simulink model "simulation_vex"  (R2024a)
settings: Solver=FixedStepAuto  StartTime=0.0  StopTime=100.0  RelTol=1e-3  EnableMultiTasking=on
libraries: vexarmcortexlib x33
settings Model: ExtModeTrigDuration=25  Creator=Mattie  LastModifiedBy=Monarch Robotics
settings SolverCC: AutoInsertRateTranBlk=on
settings OptimizationCC: EnhancedBackFolding=on  PassReuseOutputArgsAs=Individual arguments  ZeroExternalMemoryAtStartup=off  ZeroInternalMemoryAtStartup=off  MaxStackSize=64  OptimizeBlockOrder=speed  DifferentSizesBufferReuse=on  OptimizationCustomize=off  EfficientTunableParamExpr=on
settings DebuggingCC: ParameterTunabilityLossMsg=error
settings HardwareCC: ProdBitPerPointer=32  ProdBitPerSizeT=32  ProdBitPerPtrDiffT=32  ProdLargestAtomicInteger=Long  ProdLargestAtomicFloat=Double  ProdWordSize=32  ProdHWDeviceType=ARM Compatible->ARM Cortex
settings SFSimCC: MATLABDynamicMemAlloc=off
settings RTWCC: Description=Embedded Coder  SystemTargetFile=ert.tlc  HardwareBoard=ARM Cortex-based VEX Microcontroller  TLCOptions="-aInlineSetEventsForThisBaseRateFcn=TLC_FALSE -aSuppressMultiTaskScheduler=TLC_FALSE  -aRateBasedStepFcn=0"  TemplateMakefile=ert_default_tmf  Toolchain=GNU Tools for VEX ARM Cortex
settings CodeAppCC: ForceParamTrailComments=on  IgnoreCustomStorageClasses=off  OperatorAnnotations=on  SimulinkDataObjDesc=on  SFDataObjDesc=on  InsertBlockDesc=on
settings ERTTargetCC: ExtModeTransport=1  ExtModeMexFile=ext_serial_win32_comm

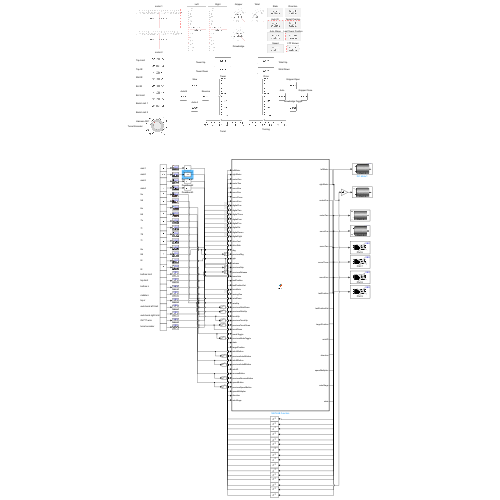
[thumbnail: Simulink's stored preview of the top-level diagram]
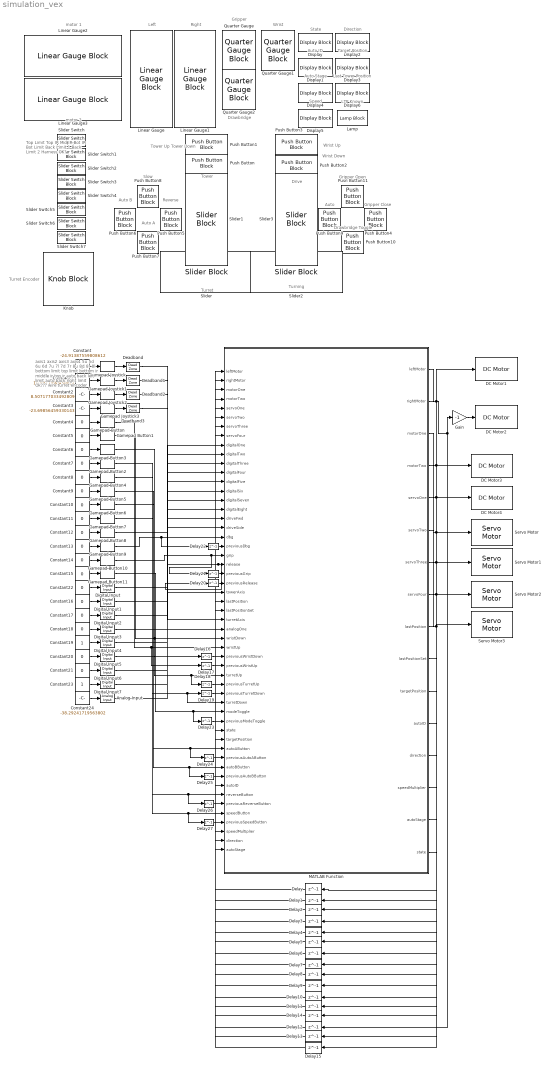
== system simulation_vex ==
  note: State
  note: Drawbridge
  note: Wrist
  note: Gripper
  note: Right
  note: Left
  note: motor 2
  note: motor 1
  note: Turret Encoder
  note: Top Limit
      |
      |
      | Top IR
      |
      |
      | Mid IR
      |
      |
      | Bot IR
      |
      |
      | Bot Limit
      |
      |
      | Back Limit 1
      |
      |
      | Back Limit 2
      |
      |
      | Harness OK?
  note: Drive
  note: Tower
  note: Turret
  note: Turning
  note: Gripper Close
  note: Gripper Open
  note: Auto
  note: Slow
  note: Reverse
  note: Auto A
  note: Auto B
  note: Wrist Down
  note: Wrist Up
  note: Tower Up
      |
      |
      | Tower Down
  note: axis1
      |
      | axis2
      |
      | axis3
      |
      |
      | axis4
      |
      | 5u
      |
      | 5d
      |
      |
      | 6u
      |
      | 6d
      |
      | 7u
      |
      |
      | 7l
      |
      | 7d
      |
      | 7r
      |
      |
      | 8u
      |
      | 8d
      |
      | 8r
      |
      |
      | 8l
      |
      | bottom limit
      |
      | top limit
      |
      | bottom ir
      |
      |
      | middle ir
      |
      | top ir
      |
      | auto back left limit
      |
      |
      | auto back right limit
      |
      | Ok??? wire
      |
      | turret encoder
  note: LTP Known
  note: Direction
  note: Target Position
  note: Auto ID
  note: Speed
  note: Auto Stage
  note: Last Tower Position
  note: Drawbridge Toggle
  Analog Input : vexarmcortexlib/Sensors/Analog Input  inChan=1  SimulationIn=on  SampleTime=0.2
  Constant : Constant  Value=-24.91387559808612
  Constant1 : Constant  Value=10.9377990430622
  Constant{4..18,20..22} (18 alike) : Constant  Value=0
  Constant19 : Constant
  Constant2 : Constant  Value=8.507177033492809
  Constant23 : Constant
  Constant24 : Constant  Value=-38.29241719563802
  Constant3 : Constant  Value=-23.69856459330143
  DC Motor1 : vexarmcortexlib/Actuators/DC Motor  motor=2  scaleFactor=1/13.5  SimulationOut=off
  DC Motor2 : vexarmcortexlib/Actuators/DC Motor  motor=3  scaleFactor=1/13.5  SimulationOut=off
  DC Motor3 : vexarmcortexlib/Actuators/DC Motor  motor=4  scaleFactor=1/13.5  SimulationOut=off
  DC Motor4 : vexarmcortexlib/Actuators/DC Motor  motor=5  scaleFactor=1/13.5  SimulationOut=off
  Deadband{,1..3} (4 alike) : DeadZone  LowerValue=-5  UpperValue=5
  Delay{,1..27} (28 alike) : Delay  DelayLength=1
  Digital Input : vexarmcortexlib/Sensors/Digital Input  inChan=1  SimulationIn=on  SampleTime=0.2
  Digital Input1 : vexarmcortexlib/Sensors/Digital Input  inChan=2  SimulationIn=on  SampleTime=0.2
  Digital Input2 : vexarmcortexlib/Sensors/Digital Input  inChan=3  SimulationIn=on  SampleTime=0.2
  Digital Input3 : vexarmcortexlib/Sensors/Digital Input  inChan=4  SimulationIn=on  SampleTime=0.2
  Digital Input4 : vexarmcortexlib/Sensors/Digital Input  inChan=5  SimulationIn=on  SampleTime=0.2
  Digital Input5 : vexarmcortexlib/Sensors/Digital Input  inChan=6  SimulationIn=on  SampleTime=0.2
  Digital Input6 : vexarmcortexlib/Sensors/Digital Input  inChan=7  SimulationIn=on  SampleTime=0.2
  Digital Input7 : vexarmcortexlib/Sensors/Digital Input  inChan=8  SimulationIn=on  SampleTime=0.2
  Display{,1..6} (7 alike) : DisplayBlock  LabelPosition=Hide  Transparency=1
  Gain : Gain  Gain=-1
  Gamepad Button : vexarmcortexlib/Gamepad/Gamepad Button  joystick=1  chan=5  button56=Up  button78=Down  SimulationIn=on  SampleTime=0.02
  Gamepad Button1 : vexarmcortexlib/Gamepad/Gamepad Button  joystick=1  chan=5  button56=Down  button78=Down  SimulationIn=on  SampleTime=0.02
  Gamepad Button10 : vexarmcortexlib/Gamepad/Gamepad Button  joystick=1  chan=8  button56=Up  button78=Right  SimulationIn=on  SampleTime=0.02
  Gamepad Button11 : vexarmcortexlib/Gamepad/Gamepad Button  joystick=1  chan=8  button56=Up  button78=Left  SimulationIn=on  SampleTime=0.02
  Gamepad Button2 : vexarmcortexlib/Gamepad/Gamepad Button  joystick=1  chan=6  button56=Down  button78=Down  SimulationIn=on  SampleTime=0.02
  Gamepad Button3 : vexarmcortexlib/Gamepad/Gamepad Button  joystick=1  chan=6  button56=Up  button78=Down  SimulationIn=on  SampleTime=0.02
  Gamepad Button4 : vexarmcortexlib/Gamepad/Gamepad Button  joystick=1  chan=7  button56=Up  button78=Up  SimulationIn=on  SampleTime=0.02
  Gamepad Button5 : vexarmcortexlib/Gamepad/Gamepad Button  joystick=1  chan=7  button56=Up  button78=Left  SimulationIn=on  SampleTime=0.02
  Gamepad Button6 : vexarmcortexlib/Gamepad/Gamepad Button  joystick=1  chan=7  button56=Up  button78=Down  SimulationIn=on  SampleTime=0.02
  Gamepad Button7 : vexarmcortexlib/Gamepad/Gamepad Button  joystick=1  chan=7  button56=Up  button78=Right  SimulationIn=on  SampleTime=0.02
  Gamepad Button8 : vexarmcortexlib/Gamepad/Gamepad Button  joystick=1  chan=8  button56=Up  button78=Up  SimulationIn=on  SampleTime=0.02
  Gamepad Button9 : vexarmcortexlib/Gamepad/Gamepad Button  joystick=1  chan=8  button56=Up  button78=Down  SimulationIn=on  SampleTime=0.02
  Gamepad Joystick : vexarmcortexlib/Gamepad/Gamepad Joystick  joystick=1  chan=1  SimulationIn=on  SampleTime=0.02
  Gamepad Joystick1 : vexarmcortexlib/Gamepad/Gamepad Joystick  joystick=1  chan=2  SimulationIn=on  SampleTime=0.02
  Gamepad Joystick2 : vexarmcortexlib/Gamepad/Gamepad Joystick  joystick=1  chan=3  SimulationIn=on  SampleTime=0.02
  Gamepad Joystick3 : vexarmcortexlib/Gamepad/Gamepad Joystick  joystick=1  chan=4  SimulationIn=on  SampleTime=0.02
  Knob : KnobBlock  LabelPosition=Hide  ScaleMin=-127  ScaleMax=127
  Lamp : LampBlock  LabelPosition=Hide
  Linear Gauge{,1..3} (4 alike) : LinearGaugeBlock  LabelPosition=Hide  ScaleMin=-127  ScaleMax=127
  MATLAB Function : MATLAB Function  TreatAsAtomicUnit=on
  Push Button{,1..11} (12 alike) : PushButtonBlock  OffValue=0.000000
  Quarter Gauge : QuarterGaugeBlock  LabelPosition=Hide  ScaleMin=-127  ScaleMax=127
  Quarter Gauge1 : QuarterGaugeBlock  LabelPosition=Hide  ScaleMin=-127  ScaleMax=127
  Quarter Gauge2 : QuarterGaugeBlock  LabelPosition=Hide  ScaleMin=-127  ScaleMax=127
  Servo Motor : vexarmcortexlib/Actuators/Servo Motor  motor=6  scaleFactor=60/127  SimulationOut=off
  Servo Motor1 : vexarmcortexlib/Actuators/Servo Motor  motor=7  scaleFactor=60/127  SimulationOut=off
  Servo Motor2 : vexarmcortexlib/Actuators/Servo Motor  motor=8  scaleFactor=60/127  SimulationOut=off
  Servo Motor3 : vexarmcortexlib/Actuators/Servo Motor  motor=9  scaleFactor=60/127  SimulationOut=off
  Slider{,1..3} (4 alike) : SliderBlock  LabelPosition=Hide  ScaleMin=-127  ScaleMax=127
  Slider Switch{,1..7} (8 alike) : SliderSwitchBlock  LabelPosition=Hide
      settings: Values={{'Off', 'On'}, [0 1]}
  wires:
  MATLAB Function/15(autoStage) -> Delay/1
  MATLAB Function/14(speedMultiplier) -> Delay1/1
  MATLAB Function/13(direction) -> Delay2/1
  MATLAB Function/12(autoID) -> Delay3/1
  MATLAB Function/11(targetPosition) -> Delay4/1
  MATLAB Function/10(lastPositionSet) -> Delay5/1
  MATLAB Function/9(lastPosition) -> Delay6/1
  MATLAB Function/8(servoFour) -> Servo Motor3/1, Delay7/1
  MATLAB Function/7(servoThree) -> Servo Motor2/1, Delay8/1
  MATLAB Function/6(servoTwo) -> Servo Motor1/1, Delay9/1
  MATLAB Function/5(servoOne) -> Servo Motor/1, Delay10/1
  MATLAB Function/1(leftMotor) -> DC Motor1/1, Delay13/1
  MATLAB Function/3(motorOne) -> DC Motor3/1, Delay14/1
  MATLAB Function/2(rightMotor) -> Gain/1, Delay12/1
  MATLAB Function/4(motorTwo) -> DC Motor4/1, Delay11/1
  Delay/1 -> MATLAB Function/53("autoStage ")
  Delay1/1 -> MATLAB Function/51("speedMultiplier ")
  Delay2/1 -> MATLAB Function/52("direction ")
  Delay3/1 -> MATLAB Function/46("autoID ")
  Delay4/1 -> MATLAB Function/41("targetPosition ")
  Delay5/1 -> MATLAB Function/27("lastPositionSet ")
  Delay13/1 -> MATLAB Function/1("leftMotor ")
  Delay12/1 -> MATLAB Function/2("rightMotor ")
  Delay14/1 -> MATLAB Function/3("motorOne ")
  Delay11/1 -> MATLAB Function/4("motorTwo ")
  Delay10/1 -> MATLAB Function/5("servoOne ")
  Delay9/1 -> MATLAB Function/6("servoTwo ")
  Delay8/1 -> MATLAB Function/7("servoThree ")
  Delay7/1 -> MATLAB Function/8("servoFour ")
  Delay6/1 -> MATLAB Function/26("lastPosition ")
  Gamepad Joystick/1 -> Deadband/1
  Gamepad Joystick1/1 -> Deadband1/1
  Gamepad Joystick2/1 -> Deadband2/1
  Gamepad Joystick3/1 -> Deadband3/1
  Gamepad Button/1 -> MATLAB Function/31(wristUp), Delay17/1
  Gamepad Button1/1 -> MATLAB Function/30(wristDown), Delay16/1
  Gamepad Button2/1 -> MATLAB Function/37(turretDown), Delay19/1
  Gamepad Button3/1 -> Delay18/1, MATLAB Function/34(turretUp)
  Digital Input/1 -> MATLAB Function/9(digitalOne)
  Digital Input1/1 -> MATLAB Function/10(digitalTwo)
  Digital Input2/1 -> MATLAB Function/11(digitalThree)
  Digital Input3/1 -> MATLAB Function/12(digitalFour)
  Digital Input4/1 -> MATLAB Function/13(digitalFive)
  Digital Input5/1 -> MATLAB Function/14(digitalSix)
  Digital Input6/1 -> MATLAB Function/15(digitalSeven)
  Digital Input7/1 -> MATLAB Function/16(digitalEight)
  Gamepad Button4/1 -> Delay27/1, MATLAB Function/49(speedButton)
  Gamepad Button7/1 -> Delay26/1, MATLAB Function/47(reverseButton)
  Gamepad Button5/1 -> Delay25/1, MATLAB Function/44(autoBButton)
  Gamepad Button6/1 -> Delay24/1, MATLAB Function/42(autoAButton)
  Gamepad Button8/1 -> Delay20/1, MATLAB Function/22(release)
  Gamepad Button10/1 -> Delay21/1, MATLAB Function/21(grip)
  Gamepad Button11/1 -> Delay23/1, MATLAB Function/38(modeToggle)
  MATLAB Function/16(state) -> Delay15/1
  Delay15/1 -> MATLAB Function/40("state ")
  Gamepad Button9/1 -> MATLAB Function/19(dbg), Delay22/1
  Analog Input/1 -> MATLAB Function/29(analogOne)
  Delay27/1 -> MATLAB Function/50(previousSpeedButton)
  Delay26/1 -> MATLAB Function/48(previousReverseButton)
  Delay25/1 -> MATLAB Function/45(previousAutoBButton)
  Delay24/1 -> MATLAB Function/43(previousAutoAButton)
  Delay23/1 -> MATLAB Function/39(previousModeToggle)
  Delay19/1 -> MATLAB Function/36(previousTurretDown)
  Delay18/1 -> MATLAB Function/35(previousTurretUp)
  Delay17/1 -> MATLAB Function/33(previousWristUp)
  Delay16/1 -> MATLAB Function/32(previousWristDown)
  Delay20/1 -> MATLAB Function/24(previousRelease)
  Delay21/1 -> MATLAB Function/23(previousGrip)
  Delay22/1 -> MATLAB Function/20(previousDbg)
  Constant/1 -> Gamepad Joystick/1
  Constant1/1 -> Gamepad Joystick1/1
  Constant2/1 -> Gamepad Joystick2/1
  Constant3/1 -> Gamepad Joystick3/1
  Constant4/1 -> Gamepad Button/1
  Constant5/1 -> Gamepad Button1/1
  Constant6/1 -> Gamepad Button3/1
  Constant7/1 -> Gamepad Button2/1
  Constant8/1 -> Gamepad Button4/1
  Constant9/1 -> Gamepad Button5/1
  Constant10/1 -> Gamepad Button6/1
  Constant11/1 -> Gamepad Button7/1
  Constant12/1 -> Gamepad Button8/1
  Constant13/1 -> Gamepad Button9/1
  Constant14/1 -> Gamepad Button10/1
  Constant15/1 -> Gamepad Button11/1
  Constant22/1 -> Digital Input/1
  Constant16/1 -> Digital Input1/1
  Constant17/1 -> Digital Input2/1
  Constant18/1 -> Digital Input3/1
  Constant19/1 -> Digital Input4/1
  Constant20/1 -> Digital Input5/1
  Constant21/1 -> Digital Input6/1
  Constant23/1 -> Digital Input7/1
  Constant24/1 -> Analog Input/1
  Gain/1 -> DC Motor2/1
  Deadband/1 -> MATLAB Function/18(driveSide)
  Deadband1/1 -> MATLAB Function/17(driveFwd)
  Deadband2/1 -> MATLAB Function/25(towerAxis)
  Deadband3/1 -> MATLAB Function/28(turretAxis)

== matlab function simulation_vex/MATLAB Function ==
  data: leftMotor input; leftMotor output; rightMotor input; motorOne input; motorTwo input; servoOne input; servoTwo input; servoThree input; servoFour input; digitalOne input; digitalTwo input; digitalThree input; digitalFour input; digitalFive input; digitalSix input; digitalSeven input; digitalEight input; driveFwd input; driveSide input; dbg input; previousDbg input; grip input; release input; previousGrip input; previousRelease input; towerAxis input; lastPosition input; lastPositionSet input; turretAxis input; analogOne input; wristDown input; wristUp input; previousWristDown input; previousWristUp input; turretUp input; previousTurretUp input; previousTurretDown input; turretDown input; modeToggle input; previousModeToggle input; state input; targetPosition input; autoAButton input; previousAutoAButton input; autoBButton input; previousAutoBButton input; autoID input; reverseButton input; previousReverseButton input; speedButton input; previousSpeedButton input; speedMultiplier input; direction input; autoStage input; rightMotor output; motorOne output; motorTwo output; servoOne output; servoTwo output; servoThree output; servoFour output; lastPosition output; lastPositionSet output; targetPosition output; autoID output; direction output; speedMultiplier output; autoStage output; state output
function [leftMotor, rightMotor, motorOne, motorTwo, servoOne, servoTwo, servoThree, servoFour, lastPosition, lastPositionSet, targetPosition, autoID, direction, speedMultiplier, autoStage, state] = robot(leftMotor, rightMotor, motorOne, motorTwo, servoOne, servoTwo, servoThree, servoFour, digitalOne, digitalTwo, digitalThree, digitalFour, digitalFive, digitalSix, digitalSeven, digitalEight, driveFwd, driveSide, dbg, previousDbg, grip, release, previousGrip, previousRelease, towerAxis, lastPosition, lastPositionSet, turretAxis, analogOne, wristDown, wristUp, previousWristDown, previousWristUp, turretUp, previousTurretUp, previousTurretDown, turretDown, modeToggle, previousModeToggle, state, targetPosition, autoAButton, previousAutoAButton, autoBButton, previousAutoBButton, autoID, reverseButton, previousReverseButton, speedButton, previousSpeedButton, speedMultiplier, direction, autoStage)
    % Constants
    DRAWBRIDGE_OPEN = 127;
    DRAWBRIDGE_CLOSE = -127;
    DRIVETRAIN_SLOW_SPEED = 0.25;
    DRIVETRAIN_FAST_SPEED = 1;
    GRIPPER_OPEN = 127;
    GRIPPER_CLOSE = -127;
    TOWER_SPEED = 100;
    TURRET_UPPER_LIMIT = 100;
    TURRET_LOWER_LIMIT = -100;
    TURRET_SLOW_ROTATE_SPEED = 40;
    TURRET_FAST_ROTATE_SPEED = 100;
    TURRET_DEAD_ZONE = 5;
    TURRET_SLOW_ZONE = 10;
    TURRET_ANGLE_CONVERSION = 1;
    WRIST_ROTATE_INCREMENT = 10;
    AUTO_TOWER_START = 0;
    AUTO_TURRET_START_A = 0;
    AUTO_TURRET_START_B = 0;
    AUTO_GRIPPER_OPEN = 0;
    AUTO_WRIST_START = 0;
    AUTO_TURRET_ROTATION = 0;
    AUTO_BACK_SPEED = 0;
    AUTO_WRIST_END = 0;
    AUTO_TOWER_MIDDLE = 0;
    AUTO_GRIPPER_CLOSE = 0;
    AUTO_TOWER_END = 0;
    AUTO_FWD_SPEED = 0;
    
    if speedMultiplier == 0
        speedMultiplier = 1;
    end

    if digitalOne == 1
        lastPosition = 0;
        lastPositionSet = 1;
    elseif digitalTwo == 1
        lastPosition = 4;
        lastPositionSet = 1;
    elseif digitalThree == 1
        lastPosition = 1;
        lastPositionSet = 1;
    elseif digitalFour == 1
        lastPosition = 2;
        lastPositionSet = 1;
    elseif digitalFive == 1
        lastPosition = 3;
        lastPositionSet = 1;
    end


    % Button states
    if digitalEight == 1
        allowedStates = 1;
    else
        allowedStates = 0;
    end

    if autoAButton == 1 && previousAutoAButton == 0
        autoID = 1;
    elseif autoBButton == 1 && previousAutoBButton == 0
        autoID = 2;
    end

    if allowedStates == 1
        if modeToggle == 0 && previousModeToggle == 1
            if state == 1
                state = 1;
                autoStage = 1;
            elseif state == 2
                state = 2;
            end
        elseif state == 0
            state = 2;
        end
    elseif allowedStates == 0
        state = 0;
    end

    if state == 0
        if previousReverseButton == 1 && reverseButton == 0
            if direction == 0
                direction = 1;
            else
                direction = 0;
            end
        end

        if direction == 1
            driveSide = driveSide * -1;
        end

        left = driveFwd + driveSide;
        right = driveFwd - driveSide;

        if previousSpeedButton == 1 && speedButton == 0
            if speedMultiplier == DRIVETRAIN_FAST_SPEED
                speedMultiplier = DRIVETRAIN_SLOW_SPEED;
            else
                speedMultiplier = DRIVETRAIN_FAST_SPEED;
            end
        end

        left = left * speedMultiplier;
        right = right * speedMultiplier;

        if direction == 1
            left = -left;
            right = -right;
        end

        % 1 is backwards, 0 is forwards
        leftMotor = left;
        rightMotor = right;

        if dbg == 1 && previousDbg == 0
            if servoThree == DRAWBRIDGE_CLOSE
                servoThree = DRAWBRIDGE_OPEN;
            else
                servoThree = DRAWBRIDGE_CLOSE;
            end
        end

        if release == 1 && previousRelease == 0
            servoOne = GRIPPER_OPEN;
        elseif grip == 1 && previousGrip == 0
            servoOne = GRIPPER_CLOSE;
        end

        if digitalOne == 1
            if towerAxis > 0
                motorTwo = towerAxis;
            else
                motorTwo = 0;
            end
        elseif digitalTwo == 1
            if towerAxis > 0
                motorTwo = towerAxis;
            else
                motorTwo = 0;
            end
        else
            motorTwo = towerAxis;
        end

        if analogOne > TURRET_UPPER_LIMIT
            if turretAxis < 0
                motorOne = turretAxis;
            else
                motorOne = 0;
            end
        elseif analogOne < TURRET_LOWER_LIMIT
            if turretAxis > 0
                motorOne = turretAxis;
            else
                motorOne = 0;
            end
        else
            motorOne = turretAxis;
        end

        if wristUp == 1 && previousWristUp == 1
            servoTwo = servoTwo + WRIST_ROTATE_INCREMENT;
        elseif wristDown == 1 && previousWristDown == 1
            servoTwo = servoTwo - WRIST_ROTATE_INCREMENT;
        end
    elseif state == 1
        if autoStage == 1
            if AUTO_TOWER_START == 1
                if digitalOne == 1
                    motorTwo = 0;
                    targetPosition = 0;
                elseif lastPosition > 0
                    motorTwo = -1 * TOWER_SPEED;
                elseif lastPosition < 0
                    motorTwo = TOWER_SPEED;
                end
            elseif AUTO_TOWER_START == 2
                if digitalThree == 1
                    motorTwo = 0;
                    targetPosition = 0;
                elseif lastPosition > 1
                    motorTwo = -1 * TOWER_SPEED;
                elseif lastPosition < 1
                    motorTwo = TOWER_SPEED;
                end
            elseif AUTO_TOWER_START == 3
                if digitalFour == 1
                    motorTwo = 0;
                    targetPosition = 0;
                elseif lastPosition > 2
                    motorTwo = -1 * TOWER_SPEED;
                elseif lastPosition < 2
                    motorTwo = TOWER_SPEED;
                end
            elseif AUTO_TOWER_START == 4
                if digitalFive == 1
                    motorTwo = 0;
                    targetPosition = 0;
                elseif lastPosition > 3
                    motorTwo = -1 * TOWER_SPEED;
                elseif lastPosition < 3
                    motorTwo = TOWER_SPEED;
                end
            elseif AUTO_TOWER_START == 5
                if digitalTwo == 1
                    motorTwo = 0;
                    targetPosition = 0;
                elseif lastPosition > 4
                    motorTwo = -1 * TOWER_SPEED;
                elseif lastPosition < 4
                    motorTwo = TOWER_SPEED;
                else
                    motorTwo = TOWER_SPEED;
                end
            end

            if autoID == 1
                AUTO_TURRET_START_A = AUTO_TURRET_START_A * TURRET_ANGLE_CONVERSION;
                if analogOne + TURRET_SLOW_ZONE > AUTO_TURRET_START_A
                    motorOne = TURRET_FAST_ROTATE_SPEED;
                elseif analogOne - TURRET_SLOW_ZONE < AUTO_TURRET_START_A
                    motorOne = -1 * TURRET_FAST_ROTATE_SPEED;
                elseif analogOne + TURRET_DEAD_ZONE > AUTO_TURRET_START_A
                    motorOne = TURRET_SLOW_ROTATE_SPEED;
                elseif analogOne - TURRET_DEAD_ZONE < AUTO_TURRET_START_A
                    motorOne = -1 * TURRET_SLOW_ROTATE_SPEED;
                else
                    motorOne = 0;
                end
            elseif autoID == 2
                AUTO_TURRET_START_B = AUTO_TURRET_START_B * TURRET_ANGLE_CONVERSION;
                if analogOne + TURRET_SLOW_ZONE > AUTO_TURRET_START_B
                    motorOne = TURRET_FAST_ROTATE_SPEED;
                elseif analogOne - TURRET_SLOW_ZONE < AUTO_TURRET_START_B
                    motorOne = -1 * TURRET_FAST_ROTATE_SPEED;
                elseif analogOne + TURRET_DEAD_ZONE > AUTO_TURRET_START_B
                    motorOne = TURRET_SLOW_ROTATE_SPEED;
                elseif analogOne - TURRET_DEAD_ZONE < AUTO_TURRET_START_B
                    motorOne = -1 * TURRET_SLOW_ROTATE_SPEED;
                else
                    motorOne = 0;
                end
            end

            servoOne = AUTO_GRIPPER_OPEN;
            servoTwo = AUTO_WRIST_START;

            if analogOne == AUTO_TURRET_ROTATION && digitalFour == 1
                autoStage = 2;
            end

        elseif autoStage == 2
            leftMotor = AUTO_BACK_SPEED;
            rightMotor = AUTO_BACK_SPEED;
            if digitalSix == 1 && digitalSeven == 1
                leftMotor = 0;
                rightMotor = 0;
                autoStage = 3;
            end

        elseif autoStage == 3
            servoTwo = AUTO_WRIST_END;
            autoStage = 4;

        elseif autoStage == 4
            % Repeat of last position setting
            if AUTO_TOWER_MIDDLE == 1
                if digitalOne == 1
                    motorTwo = 0;
                    targetPosition = 0;
                elseif lastPosition > 0
                    motorTwo = -1 * TOWER_SPEED;
                elseif lastPosition < 0
                    motorTwo = TOWER_SPEED;
                end
            elseif AUTO_TOWER_MIDDLE == 2
                if digitalThree == 1
                    motorTwo = 0;
                    targetPosition = 0;
                elseif lastPosition > 1
                    motorTwo = -1 * TOWER_SPEED;
                elseif lastPosition < 1
                    motorTwo = TOWER_SPEED;
                end
            elseif AUTO_TOWER_MIDDLE == 3
                if digitalFour == 1
                    motorTwo = 0;
                    targetPosition = 0;
                elseif lastPosition > 2
                    motorTwo = -1 * TOWER_SPEED;
                elseif lastPosition < 2
                    motorTwo = TOWER_SPEED;
                end
            elseif AUTO_TOWER_MIDDLE == 4
                if digitalFive == 1
                    motorTwo = 0;
                    targetPosition = 0;
                elseif lastPosition > 3
                    motorTwo = -1 * TOWER_SPEED;
                elseif lastPosition < 3
                    motorTwo = TOWER_SPEED;
                end
            elseif AUTO_TOWER_MIDDLE == 5
                if digitalTwo == 1
                    motorTwo = 0;
                    targetPosition = 0;
                elseif lastPosition > 4
                    motorTwo = -1 * TOWER_SPEED;
                elseif lastPosition < 4
                    motorTwo = TOWER_SPEED;
                else
                    motorTwo = TOWER_SPEED;
                end
            end

            if digitalThree == 1
                autoStage = 5;
            end

        elseif autoStage == 5
            servoOne = AUTO_GRIPPER_CLOSE;
            autoStage = 6;

        elseif autoStage == 6
            % Repeat of last position setting

            if AUTO_TOWER_END == 1
                if digitalOne == 1
                    motorTwo = 0;
                    targetPosition = 0;
                elseif lastPosition > 0
                    motorTwo = -1 * TOWER_SPEED;
                elseif lastPosition < 0
                    motorTwo = TOWER_SPEED;
                end
            elseif AUTO_TOWER_END == 2
                if digitalThree == 1
                    motorTwo = 0;
                    targetPosition = 0;
                elseif lastPosition > 1
                    motorTwo = -1 * TOWER_SPEED;
                elseif lastPosition < 1
                    motorTwo = TOWER_SPEED;
                end
            elseif AUTO_TOWER_END == 3
                if digitalFour == 1
                    motorTwo = 0;
                    targetPosition = 0;
                elseif lastPosition > 2
                    motorTwo = -1 * TOWER_SPEED;
                elseif lastPosition < 2
                    motorTwo = TOWER_SPEED;
                end
            elseif AUTO_TOWER_END == 4
                if digitalFive == 1
                    motorTwo = 0;
                    targetPosition = 0;
                elseif lastPosition > 3
                    motorTwo = -1 * TOWER_SPEED;
                elseif lastPosition < 3
                    motorTwo = TOWER_SPEED;
                end
            elseif AUTO_TOWER_END == 5
                if digitalTwo == 1
                    motorTwo = 0;
                    targetPosition = 0;
                elseif lastPosition > 4
                    motorTwo = -1 * TOWER_SPEED;
                elseif lastPosition < 4
                    motorTwo = TOWER_SPEED;
                else
                    motorTwo = TOWER_SPEED;
                end
            end
        end
    end
    if state == 2

        if previousReverseButton == 1 && reverseButton == 0
            if direction == 0
                direction = 1;
            else
                direction = 0;
            end
        end

        if direction == 1
            driveSide = driveSide * -1;
        end

        left = driveFwd + driveSide;
        right = driveFwd - driveSide;

        % Speed multiplier toggle
        if previousSpeedButton == 1 && speedButton == 0
            if speedMultiplier == 1
                speedMultiplier = 0.25;
            else
                speedMultiplier = 1;
            end
        end

        % Apply speed multiplier
        left = left * speedMultiplier;
        right = right * speedMultiplier;

        % Reverse direction if applicable
        if direction == 1
            left = -left;
            right = -right;
        end

        % Set motor speeds
        leftMotor = left;
        rightMotor = right;

        % Servo control for drawbridge
        if dbg == 1 && previousDbg == 0
            if servoThree == DRAWBRIDGE_CLOSE
                servoThree = DRAWBRIDGE_OPEN;
            else
                servoThree = DRAWBRIDGE_CLOSE;
            end
        end

        % Gripper control
        if release == 1 && previousRelease == 0
            servoOne = GRIPPER_OPEN;
        elseif grip == 1 && previousGrip == 0
            servoOne = GRIPPER_CLOSE;
        end

        % Turret movement logic
        if analogOne > TURRET_UPPER_LIMIT
            if turretAxis < 0
                motorOne = turretAxis;
            else
                motorOne = 0;
            end
        elseif analogOne < TURRET_LOWER_LIMIT
            if turretAxis > 0
                motorOne = turretAxis;
            else
                motorOne = 0;
            end
        else
            motorOne = turretAxis;
        end

        % Wrist control
        if wristUp == 1 && previousWristUp == 1
            servoTwo = servoTwo + WRIST_ROTATE_INCREMENT;
        elseif wristDown == 1 && previousWristDown == 1
            servoTwo = servoTwo - WRIST_ROTATE_INCREMENT;
        end

        % Turret position adjustment
        if turretUp == 1 && previousTurretUp == 1
            targetPosition = lastPosition + 1;
        elseif turretDown == 1 && previousTurretDown == 1
            targetPosition = lastPosition - 1;
        end

        % Tower movement based on target position
        if targetPosition == 0
            % Tower stops when in position 0
            % Tower motor control based on axis
            if digitalOne == 1 || digitalTwo == 1
                if towerAxis > 0
                    motorTwo = towerAxis;
                else
                    motorTwo = 0;
                end
            else
                motorTwo = towerAxis;
            end
        else
            % Set last position based on target position
            % Motor movement logic for tower based on target position
            if targetPosition == 1
                if digitalOne == 1
                    motorTwo = 0;
                    targetPosition = 0;
                elseif lastPosition > 0
                    motorTwo = -TOWER_SPEED;
                elseif lastPosition < 0
                    motorTwo = TOWER_SPEED;
                end
            elseif targetPosition == 2
                if digitalThree == 1
                    motorTwo = 0;
                    targetPosition = 0;
                elseif lastPosition > 1
                    motorTwo = -TOWER_SPEED;
                elseif lastPosition < 1
                    motorTwo = TOWER_SPEED;
                end
            elseif targetPosition == 3
                if digitalFour == 1
                    motorTwo = 0;
                    targetPosition = 0;
                elseif lastPosition > 2
                    motorTwo = -TOWER_SPEED;
                elseif lastPosition < 2
                    motorTwo = TOWER_SPEED;
                end
            elseif targetPosition == 4
                if digitalFive == 1
                    motorTwo = 0;
                    targetPosition = 0;
                elseif lastPosition > 3
                    motorTwo = -TOWER_SPEED;
                elseif lastPosition < 3
                    motorTwo = TOWER_SPEED;
                end
            elseif targetPosition == 5
                if digitalTwo == 1
                    motorTwo = 0;
                    targetPosition = 0;
                elseif lastPosition > 4
                    motorTwo = -TOWER_SPEED;
                elseif lastPosition < 4
                    motorTwo = TOWER_SPEED;
                else
                    motorTwo = TOWER_SPEED;
                end
            end
        end
    end
